simulink model "PendulumController"  (R2024a)
settings: Solver=FixedStepDiscrete  StartTime=0.0  StopTime=10.0  RelTol=1e-3
model workspace (MAT data in the model file):
  Ts = 0.01
  contSaturation = 10
  kd = 21
  ki = 524.5
  kp = 204.7
settings Model: Creator=sturton  LastModifiedBy=nacer

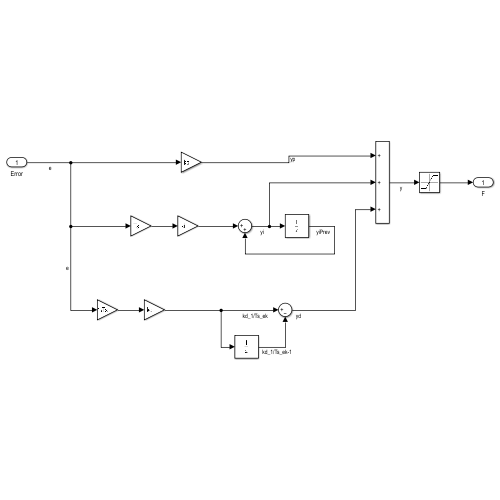
[thumbnail: Simulink's stored preview of the top-level diagram]
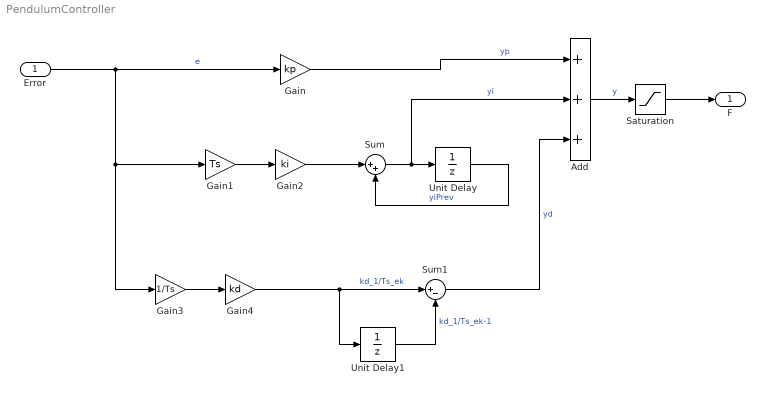
== system PendulumController ==
  Error : Inport  SampleTime=Ts
  Add : Sum  Inputs=+++
  Gain : Gain  Gain=kp
  Gain1 : Gain  Gain=Ts
  Gain2 : Gain  Gain=ki
  Gain3 : Gain  Gain=1/Ts
  Gain4 : Gain  Gain=kd
  Saturation : Saturate  UpperLimit=contSaturation  LowerLimit=-contSaturation
  Sum : Sum  Inputs=|++
  Sum1 : Sum  Inputs=|+-
  Unit Delay : UnitDelay  SampleTime=-1  HasFrameUpgradeWarning=on
  Unit Delay1 : UnitDelay  SampleTime=-1  HasFrameUpgradeWarning=on
  F : Outport
  wires:
  Error/1 -> Gain3/1, Gain1/1, Gain/1  "e"
  Gain2/1 -> Sum/1
  Gain1/1 -> Gain2/1
  Sum/1 -> Add/2, Unit Delay/1  "yi"
  Unit Delay/1 -> Sum/2  "yiPrev"
  Gain/1 -> Add/1  "yp"
  Add/1 -> Saturation/1  "y"
  Saturation/1 -> F/1
  Gain3/1 -> Gain4/1
  Gain4/1 -> Unit Delay1/1, Sum1/1  "kd_1/Ts_ek"
  Sum1/1 -> Add/3  "yd"
  Unit Delay1/1 -> Sum1/2  "kd_1/Ts_ek-1"
